simulink model "cruise_control"  (R2020b)
settings: Solver=VariableStepAuto  StartTime=0.0  StopTime=10  RelTol=1e-3
values from neighbouring files (symbols this model uses):
  b = 50    [const_declaration.m]
  m = 1000    [const_declaration.m]
settings Model: Creator=shraddha  LastModifiedBy=shraddha

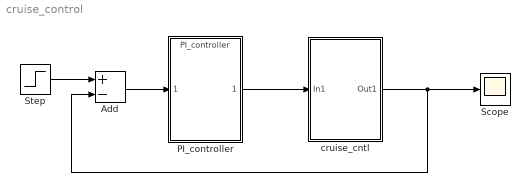
== system cruise_control ==
  Add : Sum  Inputs=+-
  PI_controller : ModelReference  ModelNameDialog=PI_controller  SimulationMode=Normal  ModelReferenceVersion=1.6
  Scope : Scope
  Step : Step  Time=0  After=u  SampleTime=0
  cruise_cntl : Subsystem
  wires:
  cruise_cntl/1(Out1) -> Add/2, Scope/1
  Step/1 -> Add/1
  Add/1 -> PI_controller/1
  PI_controller/1 -> cruise_cntl/1(In1)

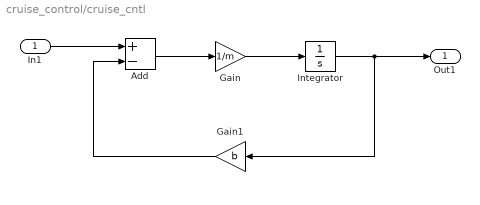
== system cruise_control/cruise_cntl ==
  In1 : Inport
  Add : Sum  Inputs=+-
  Gain : Gain  Gain=1/m
  Gain1 : Gain  Gain=b
  Integrator : Integrator
  Out1 : Outport
  wires:
  Gain/1 -> Integrator/1
  Add/1 -> Gain/1
  Gain1/1 -> Add/2
  In1/1 -> Add/1
  Integrator/1 -> Out1/1, Gain1/1
